simulink model "HARV_6DoF_turn_mdl"  (Simulink 9.3)
settings: Solver=ode45  StartTime=0.0  StopTime=100  FixedStep=0.01  MaxStep=0.01  MinStep=0.000001  RelTol=1e-3
values from neighbouring files (symbols this model uses):
  b = 37.42*0.305    (= 11.4131)    [HARV_model.m]
  cbar = 11.52*0.305    (= 3.5136)    [HARV_model.m]
  GM = [c3 0 c4 0 c2 0 0 c1 0 ... (first row only)    [HARV_model.m]
  m = 1128.09*14.5939    (= 16463.232651)    [HARV_model.m]
  S = 400*(0.305^2)    (= 37.21)    [HARV_model.m]
undefined symbols (not defined in the file or in its folder): ad, ae, airlib, B747, DT, eqm, fms, gr, hlp
libraries: simulink x1
(part 2 of 2)

== system HARV_6DoF_turn_mdl/HARV/ad/atm/Sea_level ==
  Mux : Mux  Inputs=5
  Ps_sea : Constant  Value=101325
  T_sea : Constant  Value=288.15
  g_sea : Constant  Value=9.807
  mu_sea : Constant  Value=1.789*(10^(-5))
  rho_sea : Constant  Value=1.225
  Sea Level : Outport
  wires:
  g_sea/1 -> Mux/5
  T_sea/1 -> Mux/3
  mu_sea/1 -> Mux/4
  rho_sea/1 -> Mux/1
  Ps_sea/1 -> Mux/2
  Mux/1 -> Sea Level/1

== system HARV_6DoF_turn_mdl/HARV/eqm/ODE/Eulerdot ==
  note: yeul=[psi dot; theta dot; phi dot]
  note: ueul=[x;Ftot;Mtot;yhlp]
  ueul : Inport
  Mux1 : Mux  Inputs=[29 1]
  Mux2 : Mux  Inputs=3
  phi dot : Fcn  Expr=u[4] + u[30]*u[26]
  psi dot : Fcn  Expr=(u[5]*u[28] + u[6]*u[29])/u[27]
  theta dot : Fcn  Expr=u[5]*u[29] - u[6]*u[28]
  yeul : Outport
  wires:
  Mux1/1 -> phi dot/1
  phi dot/1 -> Mux2/3
  Mux2/1 -> yeul/1
  theta dot/1 -> Mux2/2
  psi dot/1 -> Mux1/2, Mux2/1
  ueul/1 -> psi dot/1, Mux1/1, theta dot/1

== system HARV_6DoF_turn_mdl/HARV/eqm/ODE/Vabdot ==
  note: uVab=[x;Ftot;Mtot;yhlp]
  note: yVab=[V dot;alpha dot;beta dot]
  uVab : Inport
  Mux2 : Mux  Inputs=3
  V dot : Fcn  Expr=(u[13]*u[19]*u[21]+u[14]*u[22]+u[15]*u[20]*u[21])/m
  alpha dot : Fcn  Expr=(-u[13]*u[20]+u[15]*u[19])/(m*u[1]*u[21]) - u[23]*(u[4]*u[19]+u[6]*u[20]) + u[5]
  beta dot : Fcn  Expr=(-u[13]*u[19]*u[22]+u[14]*u[21]-u[15]*u[20]*u[22])/(m*u[1]) + u[4]*u[20] - u[6]*u[19]
  yVab : Outport
  wires:
  Mux2/1 -> yVab/1
  uVab/1 -> V dot/1, beta dot/1, alpha dot/1
  alpha dot/1 -> Mux2/2
  V dot/1 -> Mux2/1
  beta dot/1 -> Mux2/3

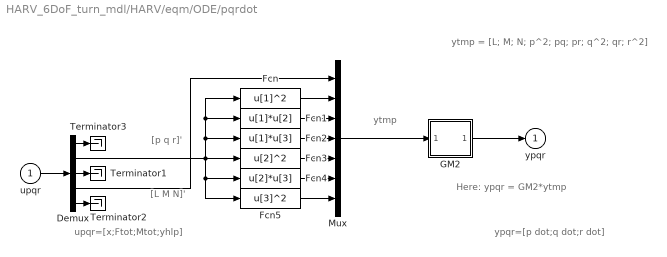
== system HARV_6DoF_turn_mdl/HARV/eqm/ODE/pqrdot ==
  note: [p q r]'
  note: [L M N]'
  note: Here: ypqr = GM2*ytmp
  note: ytmp
  note: ypqr=[p dot;q dot;r dot]
  note: upqr=[x;Ftot;Mtot;yhlp]
  note: ytmp = [L; M; N; p^2; pq; pr; q^2; qr; r^2]
  upqr : Inport
  Demux : Demux  Outputs=[3 3 9 3 11]
  Fcn : Fcn  Expr=u[1]^2
  Fcn1 : Fcn  Expr=u[1]*u[2]
  Fcn2 : Fcn  Expr=u[1]*u[3]
  Fcn3 : Fcn  Expr=u[2]^2
  Fcn4 : Fcn  Expr=u[2]*u[3]
  Fcn5 : Fcn  Expr=u[3]^2
  "GM2 " : Subsystem  mask(State Space){M=GM}
      mask prompts: M "Matrix"
      mask Display: disp('Matrix\nGain')
  Mux : Mux  Inputs=[3 1 1 1 1 1 1]
  Terminator1 : Terminator
  Terminator2 : Terminator
  Terminator3 : Terminator
  ypqr : Outport
  wires:
  upqr/1 -> Demux/1
  Demux/1 -> Terminator3/1
  Demux/5 -> Terminator2/1
  Demux/3 -> Terminator1/1
  Demux/2 -> Fcn1/1, Fcn/1, Fcn2/1, Fcn4/1, Fcn5/1, Fcn3/1
  Demux/4 -> Mux/1
  Fcn/1 -> Mux/2
  Fcn1/1 -> Mux/3
  Fcn2/1 -> Mux/4
  Fcn3/1 -> Mux/5
  Fcn4/1 -> Mux/6
  Fcn5/1 -> Mux/7
  "GM2 "/1(Out1) -> ypqr/1
  Mux/1 -> "GM2 "/1(In1)

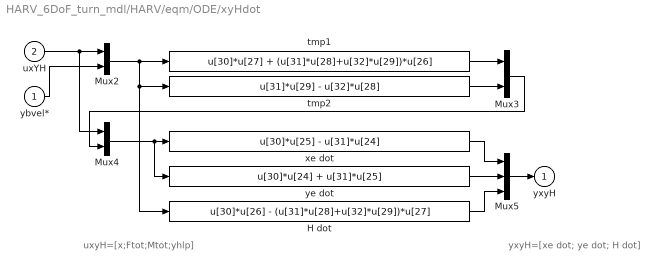
== system HARV_6DoF_turn_mdl/HARV/eqm/ODE/xyHdot ==
  note: yxyH=[xe dot; ye dot; H dot]
  note: uxyH=[x;Ftot;Mtot;yhlp]
  ybvel* : Inport
  uxYH : Inport  Port=2
  H dot : Fcn  Expr=u[30]*u[26] - (u[31]*u[28]+u[32]*u[29])*u[27]
  Mux2 : Mux  Inputs=[29 3]
  Mux3 : Mux  Inputs=2
  Mux4 : Mux  Inputs=[29 2]
  Mux5 : Mux  Inputs=3
  tmp1 : Fcn  Expr=u[30]*u[27] + (u[31]*u[28]+u[32]*u[29])*u[26]
  tmp2 : Fcn  Expr=u[31]*u[29] - u[32]*u[28]
  xe dot : Fcn  Expr=u[30]*u[25] - u[31]*u[24]
  ye dot : Fcn  Expr=u[30]*u[24] + u[31]*u[25]
  yxyH : Outport
  wires:
  tmp1/1 -> Mux3/1
  H dot/1 -> Mux5/3
  xe dot/1 -> Mux5/1
  tmp2/1 -> Mux3/2
  ye dot/1 -> Mux5/2
  Mux5/1 -> yxyH/1
  Mux4/1 -> ye dot/1, xe dot/1
  Mux2/1 -> H dot/1, tmp2/1, tmp1/1
  Mux3/1 -> Mux4/2
  ybvel*/1 -> Mux2/2
  uxYH/1 -> Mux4/1, Mux2/1

== system HARV_6DoF_turn_mdl/HARV/eqm/ODE/pqrdot/GM2  ==
  In1 : Inport
  Matrix Gain : StateSpace  A=[]  B=[]  C=[]  D=GM  InitialCondition=0
  Out1 : Outport
  wires:
  Matrix Gain/1 -> Out1/1
  In1/1 -> Matrix Gain/1
